simulink model "clusterDemo"  (Simulink 7.4)
settings: Solver=ode45  StartTime=0.0  StopTime=10.0  RelTol=1e-3
values from neighbouring files (symbols this model uses):
  A = 1    [clusterDemo.mat]
  B = [-1 -1 -1 -1 -1 -1 -1 -1 -1 -1 -1 -1 ... (21 elements, 1x21)]    [clusterDemo.mat]
  C = 1    [clusterDemo.mat]
  D = [0 0 0 0 0 0 0 0 0 0 0 0 ... (21 elements, 1x21)]    [clusterDemo.mat]
  N = 5    [clusterDemo.mat]    (also in firefliesDemo.mat = 10)
  var = 0    [clusterDemo.mat]    (also in firefliesDemo.mat = 3)
  x0 = 80    [clusterDemo.mat]
(part 2 of 4)

== system clusterDemo/Cluster/Cluster17 ==
  In1 : Inport  OutDataType=fixdt(1, 16)  OutScaling=2^0
  In2 : Inport  Port=2
  In3 : Inport  Port=3
  In4 : Inport  Port=4
  In5 : Inport  Port=5
  In6 : Inport  Port=6
  In7 : Inport  Port=7
  In8 : Inport  Port=8
  In9 : Inport  Port=9
  In10 : Inport  Port=10
  In11 : Inport  Port=11
  In12 : Inport  Port=12
  In13 : Inport  Port=13
  In14 : Inport  Port=14
  In15 : Inport  Port=15
  In16 : Inport  Port=16
  In17 : Inport  Port=17
  In18 : Inport  Port=18
  In19 : Inport  Port=19
  In20 : Inport  Port=20
  In21 : Inport  Port=21
  Mux : Mux  Inputs=21
  Scope1 : Scope
      settings: TimeRange=0.5847953216374258  YMin=-0.1657458563535892  YMax=1.21546961325967
  State-Space : StateSpace  A=A  B=B  C=C  D=D  X0=x0+var*rand(1)
  Out1 : Outport  OutDataType=fixdt(1, 16)  OutScaling=2^0
  wires:
  Mux/1 -> State-Space/1
  In1/1 -> Mux/1
  State-Space/1 -> Out1/1, Scope1/1
  In2/1 -> Mux/2
  In3/1 -> Mux/3
  In4/1 -> Mux/4
  In5/1 -> Mux/5
  In6/1 -> Mux/6
  In7/1 -> Mux/7
  In8/1 -> Mux/8
  In9/1 -> Mux/9
  In10/1 -> Mux/10
  In11/1 -> Mux/11
  In12/1 -> Mux/12
  In13/1 -> Mux/13
  In14/1 -> Mux/14
  In15/1 -> Mux/15
  In16/1 -> Mux/16
  In17/1 -> Mux/17
  In18/1 -> Mux/18
  In19/1 -> Mux/19
  In20/1 -> Mux/20
  In21/1 -> Mux/21

== system clusterDemo/Cluster/Cluster18 ==
  In1 : Inport  OutDataType=fixdt(1, 16)  OutScaling=2^0
  In2 : Inport  Port=2
  In3 : Inport  Port=3
  In4 : Inport  Port=4
  In5 : Inport  Port=5
  In6 : Inport  Port=6
  In7 : Inport  Port=7
  In8 : Inport  Port=8
  In9 : Inport  Port=9
  In10 : Inport  Port=10
  In11 : Inport  Port=11
  In12 : Inport  Port=12
  In13 : Inport  Port=13
  In14 : Inport  Port=14
  In15 : Inport  Port=15
  In16 : Inport  Port=16
  In17 : Inport  Port=17
  In18 : Inport  Port=18
  In19 : Inport  Port=19
  In20 : Inport  Port=20
  In21 : Inport  Port=21
  Mux : Mux  Inputs=21
  Scope1 : Scope
      settings: TimeRange=0.5847953216374258  YMin=-0.1657458563535892  YMax=1.21546961325967
  State-Space : StateSpace  A=A  B=B  C=C  D=D  X0=x0+var*rand(1)
  Out1 : Outport  OutDataType=fixdt(1, 16)  OutScaling=2^0
  wires:
  Mux/1 -> State-Space/1
  In1/1 -> Mux/1
  State-Space/1 -> Out1/1, Scope1/1
  In2/1 -> Mux/2
  In3/1 -> Mux/3
  In4/1 -> Mux/4
  In5/1 -> Mux/5
  In6/1 -> Mux/6
  In7/1 -> Mux/7
  In8/1 -> Mux/8
  In9/1 -> Mux/9
  In10/1 -> Mux/10
  In11/1 -> Mux/11
  In12/1 -> Mux/12
  In13/1 -> Mux/13
  In14/1 -> Mux/14
  In15/1 -> Mux/15
  In16/1 -> Mux/16
  In17/1 -> Mux/17
  In18/1 -> Mux/18
  In19/1 -> Mux/19
  In20/1 -> Mux/20
  In21/1 -> Mux/21

== system clusterDemo/Cluster/Cluster19 ==
  In1 : Inport  OutDataType=fixdt(1, 16)  OutScaling=2^0
  In2 : Inport  Port=2
  In3 : Inport  Port=3
  In4 : Inport  Port=4
  In5 : Inport  Port=5
  In6 : Inport  Port=6
  In7 : Inport  Port=7
  In8 : Inport  Port=8
  In9 : Inport  Port=9
  In10 : Inport  Port=10
  In11 : Inport  Port=11
  In12 : Inport  Port=12
  In13 : Inport  Port=13
  In14 : Inport  Port=14
  In15 : Inport  Port=15
  In16 : Inport  Port=16
  In17 : Inport  Port=17
  In18 : Inport  Port=18
  In19 : Inport  Port=19
  In20 : Inport  Port=20
  In21 : Inport  Port=21
  Mux : Mux  Inputs=21
  Scope1 : Scope
      settings: TimeRange=0.5847953216374258  YMin=-0.1657458563535892  YMax=1.21546961325967
  State-Space : StateSpace  A=A  B=B  C=C  D=D  X0=x0+var*rand(1)
  Out1 : Outport  OutDataType=fixdt(1, 16)  OutScaling=2^0
  wires:
  Mux/1 -> State-Space/1
  In1/1 -> Mux/1
  State-Space/1 -> Out1/1, Scope1/1
  In2/1 -> Mux/2
  In3/1 -> Mux/3
  In4/1 -> Mux/4
  In5/1 -> Mux/5
  In6/1 -> Mux/6
  In7/1 -> Mux/7
  In8/1 -> Mux/8
  In9/1 -> Mux/9
  In10/1 -> Mux/10
  In11/1 -> Mux/11
  In12/1 -> Mux/12
  In13/1 -> Mux/13
  In14/1 -> Mux/14
  In15/1 -> Mux/15
  In16/1 -> Mux/16
  In17/1 -> Mux/17
  In18/1 -> Mux/18
  In19/1 -> Mux/19
  In20/1 -> Mux/20
  In21/1 -> Mux/21

== system clusterDemo/Cluster/Cluster2 ==
  In1 : Inport  OutDataType=fixdt(1, 16)  OutScaling=2^0
  In2 : Inport  Port=2
  In3 : Inport  Port=3
  In4 : Inport  Port=4
  In5 : Inport  Port=5
  In6 : Inport  Port=6
  In7 : Inport  Port=7
  In8 : Inport  Port=8
  In9 : Inport  Port=9
  In10 : Inport  Port=10
  In11 : Inport  Port=11
  In12 : Inport  Port=12
  In13 : Inport  Port=13
  In14 : Inport  Port=14
  In15 : Inport  Port=15
  In16 : Inport  Port=16
  In17 : Inport  Port=17
  In18 : Inport  Port=18
  In19 : Inport  Port=19
  In20 : Inport  Port=20
  In21 : Inport  Port=21
  Mux : Mux  Inputs=21
  Scope1 : Scope
      settings: TimeRange=0.5847953216374258  YMin=-0.1657458563535892  YMax=1.21546961325967
  State-Space : StateSpace  A=A  B=B  C=C  D=D  X0=x0+var*rand(1)
  Out1 : Outport  OutDataType=fixdt(1, 16)  OutScaling=2^0
  wires:
  Mux/1 -> State-Space/1
  In1/1 -> Mux/1
  State-Space/1 -> Out1/1, Scope1/1
  In2/1 -> Mux/2
  In3/1 -> Mux/3
  In4/1 -> Mux/4
  In5/1 -> Mux/5
  In6/1 -> Mux/6
  In7/1 -> Mux/7
  In8/1 -> Mux/8
  In9/1 -> Mux/9
  In10/1 -> Mux/10
  In11/1 -> Mux/11
  In12/1 -> Mux/12
  In13/1 -> Mux/13
  In14/1 -> Mux/14
  In15/1 -> Mux/15
  In16/1 -> Mux/16
  In17/1 -> Mux/17
  In18/1 -> Mux/18
  In19/1 -> Mux/19
  In20/1 -> Mux/20
  In21/1 -> Mux/21

== system clusterDemo/Cluster/Cluster3 ==
  In1 : Inport  OutDataType=fixdt(1, 16)  OutScaling=2^0
  In2 : Inport  Port=2
  In3 : Inport  Port=3
  In4 : Inport  Port=4
  In5 : Inport  Port=5
  In6 : Inport  Port=6
  In7 : Inport  Port=7
  In8 : Inport  Port=8
  In9 : Inport  Port=9
  In10 : Inport  Port=10
  In11 : Inport  Port=11
  In12 : Inport  Port=12
  In13 : Inport  Port=13
  In14 : Inport  Port=14
  In15 : Inport  Port=15
  In16 : Inport  Port=16
  In17 : Inport  Port=17
  In18 : Inport  Port=18
  In19 : Inport  Port=19
  In20 : Inport  Port=20
  In21 : Inport  Port=21
  Mux : Mux  Inputs=21
  Scope1 : Scope
      settings: TimeRange=0.5847953216374258  YMin=-0.1657458563535892  YMax=1.21546961325967
  State-Space : StateSpace  A=A  B=B  C=C  D=D  X0=x0+var*rand(1)
  Out1 : Outport  OutDataType=fixdt(1, 16)  OutScaling=2^0
  wires:
  Mux/1 -> State-Space/1
  In1/1 -> Mux/1
  State-Space/1 -> Out1/1, Scope1/1
  In2/1 -> Mux/2
  In3/1 -> Mux/3
  In4/1 -> Mux/4
  In5/1 -> Mux/5
  In6/1 -> Mux/6
  In7/1 -> Mux/7
  In8/1 -> Mux/8
  In9/1 -> Mux/9
  In10/1 -> Mux/10
  In11/1 -> Mux/11
  In12/1 -> Mux/12
  In13/1 -> Mux/13
  In14/1 -> Mux/14
  In15/1 -> Mux/15
  In16/1 -> Mux/16
  In17/1 -> Mux/17
  In18/1 -> Mux/18
  In19/1 -> Mux/19
  In20/1 -> Mux/20
  In21/1 -> Mux/21

== system clusterDemo/Cluster/Cluster4 ==
  In1 : Inport  OutDataType=fixdt(1, 16)  OutScaling=2^0
  In2 : Inport  Port=2
  In3 : Inport  Port=3
  In4 : Inport  Port=4
  In5 : Inport  Port=5
  In6 : Inport  Port=6
  In7 : Inport  Port=7
  In8 : Inport  Port=8
  In9 : Inport  Port=9
  In10 : Inport  Port=10
  In11 : Inport  Port=11
  In12 : Inport  Port=12
  In13 : Inport  Port=13
  In14 : Inport  Port=14
  In15 : Inport  Port=15
  In16 : Inport  Port=16
  In17 : Inport  Port=17
  In18 : Inport  Port=18
  In19 : Inport  Port=19
  In20 : Inport  Port=20
  In21 : Inport  Port=21
  Mux : Mux  Inputs=21
  Scope1 : Scope
      settings: TimeRange=0.5847953216374258  YMin=-0.1657458563535892  YMax=1.21546961325967
  State-Space : StateSpace  A=A  B=B  C=C  D=D  X0=x0+var*rand(1)
  Out1 : Outport  OutDataType=fixdt(1, 16)  OutScaling=2^0
  wires:
  Mux/1 -> State-Space/1
  In1/1 -> Mux/1
  State-Space/1 -> Out1/1, Scope1/1
  In2/1 -> Mux/2
  In3/1 -> Mux/3
  In4/1 -> Mux/4
  In5/1 -> Mux/5
  In6/1 -> Mux/6
  In7/1 -> Mux/7
  In8/1 -> Mux/8
  In9/1 -> Mux/9
  In10/1 -> Mux/10
  In11/1 -> Mux/11
  In12/1 -> Mux/12
  In13/1 -> Mux/13
  In14/1 -> Mux/14
  In15/1 -> Mux/15
  In16/1 -> Mux/16
  In17/1 -> Mux/17
  In18/1 -> Mux/18
  In19/1 -> Mux/19
  In20/1 -> Mux/20
  In21/1 -> Mux/21

== system clusterDemo/Cluster/Cluster5 ==
  In1 : Inport  OutDataType=fixdt(1, 16)  OutScaling=2^0
  In2 : Inport  Port=2
  In3 : Inport  Port=3
  In4 : Inport  Port=4
  In5 : Inport  Port=5
  In6 : Inport  Port=6
  In7 : Inport  Port=7
  In8 : Inport  Port=8
  In9 : Inport  Port=9
  In10 : Inport  Port=10
  In11 : Inport  Port=11
  In12 : Inport  Port=12
  In13 : Inport  Port=13
  In14 : Inport  Port=14
  In15 : Inport  Port=15
  In16 : Inport  Port=16
  In17 : Inport  Port=17
  In18 : Inport  Port=18
  In19 : Inport  Port=19
  In20 : Inport  Port=20
  In21 : Inport  Port=21
  Mux : Mux  Inputs=21
  Scope1 : Scope
      settings: TimeRange=0.5847953216374258  YMin=-0.1657458563535892  YMax=1.21546961325967
  State-Space : StateSpace  A=A  B=B  C=C  D=D  X0=x0+var*rand(1)
  Out1 : Outport  OutDataType=fixdt(1, 16)  OutScaling=2^0
  wires:
  Mux/1 -> State-Space/1
  In1/1 -> Mux/1
  State-Space/1 -> Out1/1, Scope1/1
  In2/1 -> Mux/2
  In3/1 -> Mux/3
  In4/1 -> Mux/4
  In5/1 -> Mux/5
  In6/1 -> Mux/6
  In7/1 -> Mux/7
  In8/1 -> Mux/8
  In9/1 -> Mux/9
  In10/1 -> Mux/10
  In11/1 -> Mux/11
  In12/1 -> Mux/12
  In13/1 -> Mux/13
  In14/1 -> Mux/14
  In15/1 -> Mux/15
  In16/1 -> Mux/16
  In17/1 -> Mux/17
  In18/1 -> Mux/18
  In19/1 -> Mux/19
  In20/1 -> Mux/20
  In21/1 -> Mux/21

== system clusterDemo/Cluster/Cluster6 ==
  In1 : Inport  OutDataType=fixdt(1, 16)  OutScaling=2^0
  In2 : Inport  Port=2
  In3 : Inport  Port=3
  In4 : Inport  Port=4
  In5 : Inport  Port=5
  In6 : Inport  Port=6
  In7 : Inport  Port=7
  In8 : Inport  Port=8
  In9 : Inport  Port=9
  In10 : Inport  Port=10
  In11 : Inport  Port=11
  In12 : Inport  Port=12
  In13 : Inport  Port=13
  In14 : Inport  Port=14
  In15 : Inport  Port=15
  In16 : Inport  Port=16
  In17 : Inport  Port=17
  In18 : Inport  Port=18
  In19 : Inport  Port=19
  In20 : Inport  Port=20
  In21 : Inport  Port=21
  Mux : Mux  Inputs=21
  Scope1 : Scope
      settings: TimeRange=0.5847953216374258  YMin=-0.1657458563535892  YMax=1.21546961325967
  State-Space : StateSpace  A=A  B=B  C=C  D=D  X0=x0+var*rand(1)
  Out1 : Outport  OutDataType=fixdt(1, 16)  OutScaling=2^0
  wires:
  Mux/1 -> State-Space/1
  In1/1 -> Mux/1
  State-Space/1 -> Out1/1, Scope1/1
  In2/1 -> Mux/2
  In3/1 -> Mux/3
  In4/1 -> Mux/4
  In5/1 -> Mux/5
  In6/1 -> Mux/6
  In7/1 -> Mux/7
  In8/1 -> Mux/8
  In9/1 -> Mux/9
  In10/1 -> Mux/10
  In11/1 -> Mux/11
  In12/1 -> Mux/12
  In13/1 -> Mux/13
  In14/1 -> Mux/14
  In15/1 -> Mux/15
  In16/1 -> Mux/16
  In17/1 -> Mux/17
  In18/1 -> Mux/18
  In19/1 -> Mux/19
  In20/1 -> Mux/20
  In21/1 -> Mux/21

== system clusterDemo/Cluster/Cluster7 ==
  In1 : Inport  OutDataType=fixdt(1, 16)  OutScaling=2^0
  In2 : Inport  Port=2
  In3 : Inport  Port=3
  In4 : Inport  Port=4
  In5 : Inport  Port=5
  In6 : Inport  Port=6
  In7 : Inport  Port=7
  In8 : Inport  Port=8
  In9 : Inport  Port=9
  In10 : Inport  Port=10
  In11 : Inport  Port=11
  In12 : Inport  Port=12
  In13 : Inport  Port=13
  In14 : Inport  Port=14
  In15 : Inport  Port=15
  In16 : Inport  Port=16
  In17 : Inport  Port=17
  In18 : Inport  Port=18
  In19 : Inport  Port=19
  In20 : Inport  Port=20
  In21 : Inport  Port=21
  Mux : Mux  Inputs=21
  Scope1 : Scope
      settings: TimeRange=0.5847953216374258  YMin=-0.1657458563535892  YMax=1.21546961325967
  State-Space : StateSpace  A=A  B=B  C=C  D=D  X0=x0+var*rand(1)
  Out1 : Outport  OutDataType=fixdt(1, 16)  OutScaling=2^0
  wires:
  Mux/1 -> State-Space/1
  In1/1 -> Mux/1
  State-Space/1 -> Out1/1, Scope1/1
  In2/1 -> Mux/2
  In3/1 -> Mux/3
  In4/1 -> Mux/4
  In5/1 -> Mux/5
  In6/1 -> Mux/6
  In7/1 -> Mux/7
  In8/1 -> Mux/8
  In9/1 -> Mux/9
  In10/1 -> Mux/10
  In11/1 -> Mux/11
  In12/1 -> Mux/12
  In13/1 -> Mux/13
  In14/1 -> Mux/14
  In15/1 -> Mux/15
  In16/1 -> Mux/16
  In17/1 -> Mux/17
  In18/1 -> Mux/18
  In19/1 -> Mux/19
  In20/1 -> Mux/20
  In21/1 -> Mux/21

== system clusterDemo/Cluster/Cluster8 ==
  In1 : Inport  OutDataType=fixdt(1, 16)  OutScaling=2^0
  In2 : Inport  Port=2
  In3 : Inport  Port=3
  In4 : Inport  Port=4
  In5 : Inport  Port=5
  In6 : Inport  Port=6
  In7 : Inport  Port=7
  In8 : Inport  Port=8
  In9 : Inport  Port=9
  In10 : Inport  Port=10
  In11 : Inport  Port=11
  In12 : Inport  Port=12
  In13 : Inport  Port=13
  In14 : Inport  Port=14
  In15 : Inport  Port=15
  In16 : Inport  Port=16
  In17 : Inport  Port=17
  In18 : Inport  Port=18
  In19 : Inport  Port=19
  In20 : Inport  Port=20
  In21 : Inport  Port=21
  Mux : Mux  Inputs=21
  Scope1 : Scope
      settings: TimeRange=0.5847953216374258  YMin=-0.1657458563535892  YMax=1.21546961325967
  State-Space : StateSpace  A=A  B=B  C=C  D=D  X0=x0+var*rand(1)
  Out1 : Outport  OutDataType=fixdt(1, 16)  OutScaling=2^0
  wires:
  Mux/1 -> State-Space/1
  In1/1 -> Mux/1
  State-Space/1 -> Out1/1, Scope1/1
  In2/1 -> Mux/2
  In3/1 -> Mux/3
  In4/1 -> Mux/4
  In5/1 -> Mux/5
  In6/1 -> Mux/6
  In7/1 -> Mux/7
  In8/1 -> Mux/8
  In9/1 -> Mux/9
  In10/1 -> Mux/10
  In11/1 -> Mux/11
  In12/1 -> Mux/12
  In13/1 -> Mux/13
  In14/1 -> Mux/14
  In15/1 -> Mux/15
  In16/1 -> Mux/16
  In17/1 -> Mux/17
  In18/1 -> Mux/18
  In19/1 -> Mux/19
  In20/1 -> Mux/20
  In21/1 -> Mux/21

== system clusterDemo/Cluster/Cluster9 ==
  In1 : Inport  OutDataType=fixdt(1, 16)  OutScaling=2^0
  In2 : Inport  Port=2
  In3 : Inport  Port=3
  In4 : Inport  Port=4
  In5 : Inport  Port=5
  In6 : Inport  Port=6
  In7 : Inport  Port=7
  In8 : Inport  Port=8
  In9 : Inport  Port=9
  In10 : Inport  Port=10
  In11 : Inport  Port=11
  In12 : Inport  Port=12
  In13 : Inport  Port=13
  In14 : Inport  Port=14
  In15 : Inport  Port=15
  In16 : Inport  Port=16
  In17 : Inport  Port=17
  In18 : Inport  Port=18
  In19 : Inport  Port=19
  In20 : Inport  Port=20
  In21 : Inport  Port=21
  Mux : Mux  Inputs=21
  Scope1 : Scope
      settings: TimeRange=0.5847953216374258  YMin=-0.1657458563535892  YMax=1.21546961325967
  State-Space : StateSpace  A=A  B=B  C=C  D=D  X0=x0+var*rand(1)
  Out1 : Outport  OutDataType=fixdt(1, 16)  OutScaling=2^0
  wires:
  Mux/1 -> State-Space/1
  In1/1 -> Mux/1
  State-Space/1 -> Out1/1, Scope1/1
  In2/1 -> Mux/2
  In3/1 -> Mux/3
  In4/1 -> Mux/4
  In5/1 -> Mux/5
  In6/1 -> Mux/6
  In7/1 -> Mux/7
  In8/1 -> Mux/8
  In9/1 -> Mux/9
  In10/1 -> Mux/10
  In11/1 -> Mux/11
  In12/1 -> Mux/12
  In13/1 -> Mux/13
  In14/1 -> Mux/14
  In15/1 -> Mux/15
  In16/1 -> Mux/16
  In17/1 -> Mux/17
  In18/1 -> Mux/18
  In19/1 -> Mux/19
  In20/1 -> Mux/20
  In21/1 -> Mux/21

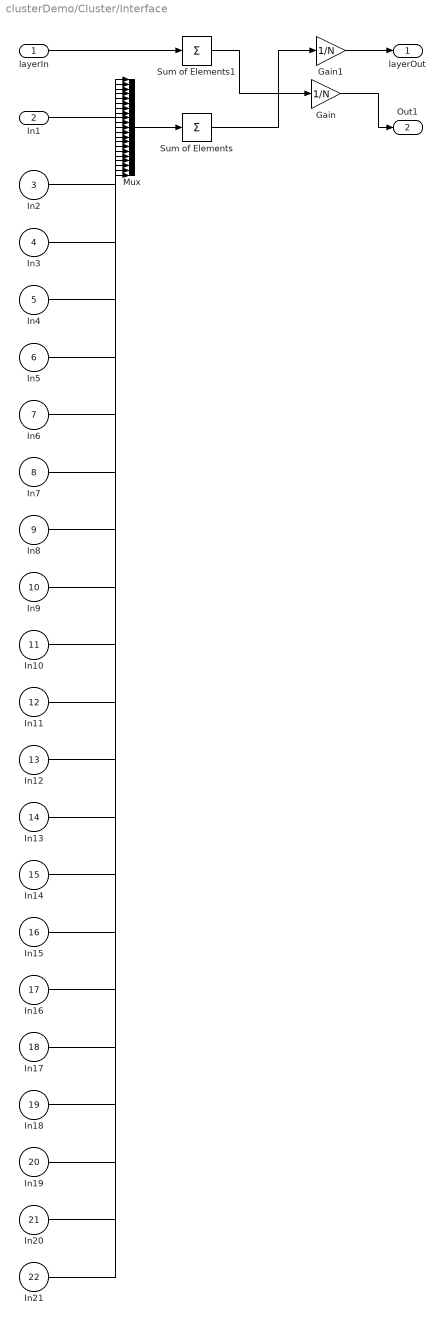
== system clusterDemo/Cluster/Interface ==
  layerIn : Inport  OutDataType=fixdt(1, 16)  OutScaling=2^0
  In1 : Inport  Port=2  OutDataType=fixdt(1, 16)  OutScaling=2^0
  In2 : Inport  Port=3
  In3 : Inport  Port=4
  In4 : Inport  Port=5
  In5 : Inport  Port=6
  In6 : Inport  Port=7
  In7 : Inport  Port=8
  In8 : Inport  Port=9
  In9 : Inport  Port=10
  In10 : Inport  Port=11
  In11 : Inport  Port=12
  In12 : Inport  Port=13
  In13 : Inport  Port=14
  In14 : Inport  Port=15
  In15 : Inport  Port=16
  In16 : Inport  Port=17
  In17 : Inport  Port=18
  In18 : Inport  Port=19
  In19 : Inport  Port=20
  In20 : Inport  Port=21
  In21 : Inport  Port=22
  Gain : Gain  Gain=1/N  ParameterDataType=fixdt(1, 16)  ParameterScaling=2^0  OutDataType=fixdt(1, 16)  OutScaling=2^0
  Gain1 : Gain  Gain=1/N  ParameterDataType=fixdt(1, 16)  ParameterScaling=2^0  OutDataType=fixdt(1, 16)  OutScaling=2^0
  Mux : Mux  Inputs=21
  Sum of Elements : Sum  Inputs=+  OutDataType=fixdt(1, 16)  OutScaling=2^-10
  Sum of Elements1 : Sum  Inputs=+  OutDataType=fixdt(1, 16)  OutScaling=2^-10
  layerOut : Outport  OutDataType=fixdt(1, 16)  OutScaling=2^0
  Out1 : Outport  Port=2  OutDataType=fixdt(1, 16)  OutScaling=2^0
  wires:
  Mux/1 -> Sum of Elements/1
  In1/1 -> Mux/1
  Sum of Elements/1 -> Gain1/1
  layerIn/1 -> Sum of Elements1/1
  Sum of Elements1/1 -> Gain/1
  Gain/1 -> Out1/1
  Gain1/1 -> layerOut/1
  In2/1 -> Mux/2
  In3/1 -> Mux/3
  In4/1 -> Mux/4
  In5/1 -> Mux/5
  In6/1 -> Mux/6
  In7/1 -> Mux/7
  In8/1 -> Mux/8
  In9/1 -> Mux/9
  In10/1 -> Mux/10
  In11/1 -> Mux/11
  In12/1 -> Mux/12
  In13/1 -> Mux/13
  In14/1 -> Mux/14
  In15/1 -> Mux/15
  In16/1 -> Mux/16
  In17/1 -> Mux/17
  In18/1 -> Mux/18
  In19/1 -> Mux/19
  In20/1 -> Mux/20
  In21/1 -> Mux/21

== system clusterDemo/Cluster1/Cluster ==
  In1 : Inport  OutDataType=fixdt(1, 16)  OutScaling=2^0
  In2 : Inport  Port=2
  In3 : Inport  Port=3
  In4 : Inport  Port=4
  In5 : Inport  Port=5
  In6 : Inport  Port=6
  In7 : Inport  Port=7
  In8 : Inport  Port=8
  In9 : Inport  Port=9
  In10 : Inport  Port=10
  In11 : Inport  Port=11
  In12 : Inport  Port=12
  In13 : Inport  Port=13
  In14 : Inport  Port=14
  In15 : Inport  Port=15
  In16 : Inport  Port=16
  In17 : Inport  Port=17
  In18 : Inport  Port=18
  In19 : Inport  Port=19
  In20 : Inport  Port=20
  In21 : Inport  Port=21
  Mux : Mux  Inputs=21
  Scope1 : Scope
      settings: TimeRange=0.5847953216374258  YMin=-0.1657458563535892  YMax=1.21546961325967
  State-Space : StateSpace  A=A  B=B  C=C  D=D  X0=x0+var*rand(1)
  Out1 : Outport  OutDataType=fixdt(1, 16)  OutScaling=2^0
  wires:
  Mux/1 -> State-Space/1
  In1/1 -> Mux/1
  State-Space/1 -> Out1/1, Scope1/1
  In2/1 -> Mux/2
  In3/1 -> Mux/3
  In4/1 -> Mux/4
  In5/1 -> Mux/5
  In6/1 -> Mux/6
  In7/1 -> Mux/7
  In8/1 -> Mux/8
  In9/1 -> Mux/9
  In10/1 -> Mux/10
  In11/1 -> Mux/11
  In12/1 -> Mux/12
  In13/1 -> Mux/13
  In14/1 -> Mux/14
  In15/1 -> Mux/15
  In16/1 -> Mux/16
  In17/1 -> Mux/17
  In18/1 -> Mux/18
  In19/1 -> Mux/19
  In20/1 -> Mux/20
  In21/1 -> Mux/21

== system clusterDemo/Cluster1/Cluster1 ==
  In1 : Inport  OutDataType=fixdt(1, 16)  OutScaling=2^0
  In2 : Inport  Port=2
  In3 : Inport  Port=3
  In4 : Inport  Port=4
  In5 : Inport  Port=5
  In6 : Inport  Port=6
  In7 : Inport  Port=7
  In8 : Inport  Port=8
  In9 : Inport  Port=9
  In10 : Inport  Port=10
  In11 : Inport  Port=11
  In12 : Inport  Port=12
  In13 : Inport  Port=13
  In14 : Inport  Port=14
  In15 : Inport  Port=15
  In16 : Inport  Port=16
  In17 : Inport  Port=17
  In18 : Inport  Port=18
  In19 : Inport  Port=19
  In20 : Inport  Port=20
  In21 : Inport  Port=21
  Mux : Mux  Inputs=21
  Scope1 : Scope
      settings: TimeRange=0.5847953216374258  YMin=-0.1657458563535892  YMax=1.21546961325967
  State-Space : StateSpace  A=A  B=B  C=C  D=D  X0=x0+var*rand(1)
  Out1 : Outport  OutDataType=fixdt(1, 16)  OutScaling=2^0
  wires:
  Mux/1 -> State-Space/1
  In1/1 -> Mux/1
  State-Space/1 -> Out1/1, Scope1/1
  In2/1 -> Mux/2
  In3/1 -> Mux/3
  In4/1 -> Mux/4
  In5/1 -> Mux/5
  In6/1 -> Mux/6
  In7/1 -> Mux/7
  In8/1 -> Mux/8
  In9/1 -> Mux/9
  In10/1 -> Mux/10
  In11/1 -> Mux/11
  In12/1 -> Mux/12
  In13/1 -> Mux/13
  In14/1 -> Mux/14
  In15/1 -> Mux/15
  In16/1 -> Mux/16
  In17/1 -> Mux/17
  In18/1 -> Mux/18
  In19/1 -> Mux/19
  In20/1 -> Mux/20
  In21/1 -> Mux/21

== system clusterDemo/Cluster1/Cluster10 ==
  In1 : Inport  OutDataType=fixdt(1, 16)  OutScaling=2^0
  In2 : Inport  Port=2
  In3 : Inport  Port=3
  In4 : Inport  Port=4
  In5 : Inport  Port=5
  In6 : Inport  Port=6
  In7 : Inport  Port=7
  In8 : Inport  Port=8
  In9 : Inport  Port=9
  In10 : Inport  Port=10
  In11 : Inport  Port=11
  In12 : Inport  Port=12
  In13 : Inport  Port=13
  In14 : Inport  Port=14
  In15 : Inport  Port=15
  In16 : Inport  Port=16
  In17 : Inport  Port=17
  In18 : Inport  Port=18
  In19 : Inport  Port=19
  In20 : Inport  Port=20
  In21 : Inport  Port=21
  Mux : Mux  Inputs=21
  Scope1 : Scope
      settings: TimeRange=0.5847953216374258  YMin=-0.1657458563535892  YMax=1.21546961325967
  State-Space : StateSpace  A=A  B=B  C=C  D=D  X0=x0+var*rand(1)
  Out1 : Outport  OutDataType=fixdt(1, 16)  OutScaling=2^0
  wires:
  Mux/1 -> State-Space/1
  In1/1 -> Mux/1
  State-Space/1 -> Out1/1, Scope1/1
  In2/1 -> Mux/2
  In3/1 -> Mux/3
  In4/1 -> Mux/4
  In5/1 -> Mux/5
  In6/1 -> Mux/6
  In7/1 -> Mux/7
  In8/1 -> Mux/8
  In9/1 -> Mux/9
  In10/1 -> Mux/10
  In11/1 -> Mux/11
  In12/1 -> Mux/12
  In13/1 -> Mux/13
  In14/1 -> Mux/14
  In15/1 -> Mux/15
  In16/1 -> Mux/16
  In17/1 -> Mux/17
  In18/1 -> Mux/18
  In19/1 -> Mux/19
  In20/1 -> Mux/20
  In21/1 -> Mux/21

== system clusterDemo/Cluster1/Cluster11 ==
  In1 : Inport  OutDataType=fixdt(1, 16)  OutScaling=2^0
  In2 : Inport  Port=2
  In3 : Inport  Port=3
  In4 : Inport  Port=4
  In5 : Inport  Port=5
  In6 : Inport  Port=6
  In7 : Inport  Port=7
  In8 : Inport  Port=8
  In9 : Inport  Port=9
  In10 : Inport  Port=10
  In11 : Inport  Port=11
  In12 : Inport  Port=12
  In13 : Inport  Port=13
  In14 : Inport  Port=14
  In15 : Inport  Port=15
  In16 : Inport  Port=16
  In17 : Inport  Port=17
  In18 : Inport  Port=18
  In19 : Inport  Port=19
  In20 : Inport  Port=20
  In21 : Inport  Port=21
  Mux : Mux  Inputs=21
  Scope1 : Scope
      settings: TimeRange=0.5847953216374258  YMin=-0.1657458563535892  YMax=1.21546961325967
  State-Space : StateSpace  A=A  B=B  C=C  D=D  X0=x0+var*rand(1)
  Out1 : Outport  OutDataType=fixdt(1, 16)  OutScaling=2^0
  wires:
  Mux/1 -> State-Space/1
  In1/1 -> Mux/1
  State-Space/1 -> Out1/1, Scope1/1
  In2/1 -> Mux/2
  In3/1 -> Mux/3
  In4/1 -> Mux/4
  In5/1 -> Mux/5
  In6/1 -> Mux/6
  In7/1 -> Mux/7
  In8/1 -> Mux/8
  In9/1 -> Mux/9
  In10/1 -> Mux/10
  In11/1 -> Mux/11
  In12/1 -> Mux/12
  In13/1 -> Mux/13
  In14/1 -> Mux/14
  In15/1 -> Mux/15
  In16/1 -> Mux/16
  In17/1 -> Mux/17
  In18/1 -> Mux/18
  In19/1 -> Mux/19
  In20/1 -> Mux/20
  In21/1 -> Mux/21

== system clusterDemo/Cluster1/Cluster12 ==
  In1 : Inport  OutDataType=fixdt(1, 16)  OutScaling=2^0
  In2 : Inport  Port=2
  In3 : Inport  Port=3
  In4 : Inport  Port=4
  In5 : Inport  Port=5
  In6 : Inport  Port=6
  In7 : Inport  Port=7
  In8 : Inport  Port=8
  In9 : Inport  Port=9
  In10 : Inport  Port=10
  In11 : Inport  Port=11
  In12 : Inport  Port=12
  In13 : Inport  Port=13
  In14 : Inport  Port=14
  In15 : Inport  Port=15
  In16 : Inport  Port=16
  In17 : Inport  Port=17
  In18 : Inport  Port=18
  In19 : Inport  Port=19
  In20 : Inport  Port=20
  In21 : Inport  Port=21
  Mux : Mux  Inputs=21
  Scope1 : Scope
      settings: TimeRange=0.5847953216374258  YMin=-0.1657458563535892  YMax=1.21546961325967
  State-Space : StateSpace  A=A  B=B  C=C  D=D  X0=x0+var*rand(1)
  Out1 : Outport  OutDataType=fixdt(1, 16)  OutScaling=2^0
  wires:
  Mux/1 -> State-Space/1
  In1/1 -> Mux/1
  State-Space/1 -> Out1/1, Scope1/1
  In2/1 -> Mux/2
  In3/1 -> Mux/3
  In4/1 -> Mux/4
  In5/1 -> Mux/5
  In6/1 -> Mux/6
  In7/1 -> Mux/7
  In8/1 -> Mux/8
  In9/1 -> Mux/9
  In10/1 -> Mux/10
  In11/1 -> Mux/11
  In12/1 -> Mux/12
  In13/1 -> Mux/13
  In14/1 -> Mux/14
  In15/1 -> Mux/15
  In16/1 -> Mux/16
  In17/1 -> Mux/17
  In18/1 -> Mux/18
  In19/1 -> Mux/19
  In20/1 -> Mux/20
  In21/1 -> Mux/21

== system clusterDemo/Cluster1/Cluster13 ==
  In1 : Inport  OutDataType=fixdt(1, 16)  OutScaling=2^0
  In2 : Inport  Port=2
  In3 : Inport  Port=3
  In4 : Inport  Port=4
  In5 : Inport  Port=5
  In6 : Inport  Port=6
  In7 : Inport  Port=7
  In8 : Inport  Port=8
  In9 : Inport  Port=9
  In10 : Inport  Port=10
  In11 : Inport  Port=11
  In12 : Inport  Port=12
  In13 : Inport  Port=13
  In14 : Inport  Port=14
  In15 : Inport  Port=15
  In16 : Inport  Port=16
  In17 : Inport  Port=17
  In18 : Inport  Port=18
  In19 : Inport  Port=19
  In20 : Inport  Port=20
  In21 : Inport  Port=21
  Mux : Mux  Inputs=21
  Scope1 : Scope
      settings: TimeRange=0.5847953216374258  YMin=-0.1657458563535892  YMax=1.21546961325967
  State-Space : StateSpace  A=A  B=B  C=C  D=D  X0=x0+var*rand(1)
  Out1 : Outport  OutDataType=fixdt(1, 16)  OutScaling=2^0
  wires:
  Mux/1 -> State-Space/1
  In1/1 -> Mux/1
  State-Space/1 -> Out1/1, Scope1/1
  In2/1 -> Mux/2
  In3/1 -> Mux/3
  In4/1 -> Mux/4
  In5/1 -> Mux/5
  In6/1 -> Mux/6
  In7/1 -> Mux/7
  In8/1 -> Mux/8
  In9/1 -> Mux/9
  In10/1 -> Mux/10
  In11/1 -> Mux/11
  In12/1 -> Mux/12
  In13/1 -> Mux/13
  In14/1 -> Mux/14
  In15/1 -> Mux/15
  In16/1 -> Mux/16
  In17/1 -> Mux/17
  In18/1 -> Mux/18
  In19/1 -> Mux/19
  In20/1 -> Mux/20
  In21/1 -> Mux/21

== system clusterDemo/Cluster1/Cluster14 ==
  In1 : Inport  OutDataType=fixdt(1, 16)  OutScaling=2^0
  In2 : Inport  Port=2
  In3 : Inport  Port=3
  In4 : Inport  Port=4
  In5 : Inport  Port=5
  In6 : Inport  Port=6
  In7 : Inport  Port=7
  In8 : Inport  Port=8
  In9 : Inport  Port=9
  In10 : Inport  Port=10
  In11 : Inport  Port=11
  In12 : Inport  Port=12
  In13 : Inport  Port=13
  In14 : Inport  Port=14
  In15 : Inport  Port=15
  In16 : Inport  Port=16
  In17 : Inport  Port=17
  In18 : Inport  Port=18
  In19 : Inport  Port=19
  In20 : Inport  Port=20
  In21 : Inport  Port=21
  Mux : Mux  Inputs=21
  Scope1 : Scope
      settings: TimeRange=0.5847953216374258  YMin=-0.1657458563535892  YMax=1.21546961325967
  State-Space : StateSpace  A=A  B=B  C=C  D=D  X0=x0+var*rand(1)
  Out1 : Outport  OutDataType=fixdt(1, 16)  OutScaling=2^0
  wires:
  Mux/1 -> State-Space/1
  In1/1 -> Mux/1
  State-Space/1 -> Out1/1, Scope1/1
  In2/1 -> Mux/2
  In3/1 -> Mux/3
  In4/1 -> Mux/4
  In5/1 -> Mux/5
  In6/1 -> Mux/6
  In7/1 -> Mux/7
  In8/1 -> Mux/8
  In9/1 -> Mux/9
  In10/1 -> Mux/10
  In11/1 -> Mux/11
  In12/1 -> Mux/12
  In13/1 -> Mux/13
  In14/1 -> Mux/14
  In15/1 -> Mux/15
  In16/1 -> Mux/16
  In17/1 -> Mux/17
  In18/1 -> Mux/18
  In19/1 -> Mux/19
  In20/1 -> Mux/20
  In21/1 -> Mux/21

== system clusterDemo/Cluster1/Cluster15 ==
  In1 : Inport  OutDataType=fixdt(1, 16)  OutScaling=2^0
  In2 : Inport  Port=2
  In3 : Inport  Port=3
  In4 : Inport  Port=4
  In5 : Inport  Port=5
  In6 : Inport  Port=6
  In7 : Inport  Port=7
  In8 : Inport  Port=8
  In9 : Inport  Port=9
  In10 : Inport  Port=10
  In11 : Inport  Port=11
  In12 : Inport  Port=12
  In13 : Inport  Port=13
  In14 : Inport  Port=14
  In15 : Inport  Port=15
  In16 : Inport  Port=16
  In17 : Inport  Port=17
  In18 : Inport  Port=18
  In19 : Inport  Port=19
  In20 : Inport  Port=20
  In21 : Inport  Port=21
  Mux : Mux  Inputs=21
  Scope1 : Scope
      settings: TimeRange=0.5847953216374258  YMin=-0.1657458563535892  YMax=1.21546961325967
  State-Space : StateSpace  A=A  B=B  C=C  D=D  X0=x0+var*rand(1)
  Out1 : Outport  OutDataType=fixdt(1, 16)  OutScaling=2^0
  wires:
  Mux/1 -> State-Space/1
  In1/1 -> Mux/1
  State-Space/1 -> Out1/1, Scope1/1
  In2/1 -> Mux/2
  In3/1 -> Mux/3
  In4/1 -> Mux/4
  In5/1 -> Mux/5
  In6/1 -> Mux/6
  In7/1 -> Mux/7
  In8/1 -> Mux/8
  In9/1 -> Mux/9
  In10/1 -> Mux/10
  In11/1 -> Mux/11
  In12/1 -> Mux/12
  In13/1 -> Mux/13
  In14/1 -> Mux/14
  In15/1 -> Mux/15
  In16/1 -> Mux/16
  In17/1 -> Mux/17
  In18/1 -> Mux/18
  In19/1 -> Mux/19
  In20/1 -> Mux/20
  In21/1 -> Mux/21

== system clusterDemo/Cluster1/Cluster16 ==
  In1 : Inport  OutDataType=fixdt(1, 16)  OutScaling=2^0
  In2 : Inport  Port=2
  In3 : Inport  Port=3
  In4 : Inport  Port=4
  In5 : Inport  Port=5
  In6 : Inport  Port=6
  In7 : Inport  Port=7
  In8 : Inport  Port=8
  In9 : Inport  Port=9
  In10 : Inport  Port=10
  In11 : Inport  Port=11
  In12 : Inport  Port=12
  In13 : Inport  Port=13
  In14 : Inport  Port=14
  In15 : Inport  Port=15
  In16 : Inport  Port=16
  In17 : Inport  Port=17
  In18 : Inport  Port=18
  In19 : Inport  Port=19
  In20 : Inport  Port=20
  In21 : Inport  Port=21
  Mux : Mux  Inputs=21
  Scope1 : Scope
      settings: TimeRange=0.5847953216374258  YMin=-0.1657458563535892  YMax=1.21546961325967
  State-Space : StateSpace  A=A  B=B  C=C  D=D  X0=x0+var*rand(1)
  Out1 : Outport  OutDataType=fixdt(1, 16)  OutScaling=2^0
  wires:
  Mux/1 -> State-Space/1
  In1/1 -> Mux/1
  State-Space/1 -> Out1/1, Scope1/1
  In2/1 -> Mux/2
  In3/1 -> Mux/3
  In4/1 -> Mux/4
  In5/1 -> Mux/5
  In6/1 -> Mux/6
  In7/1 -> Mux/7
  In8/1 -> Mux/8
  In9/1 -> Mux/9
  In10/1 -> Mux/10
  In11/1 -> Mux/11
  In12/1 -> Mux/12
  In13/1 -> Mux/13
  In14/1 -> Mux/14
  In15/1 -> Mux/15
  In16/1 -> Mux/16
  In17/1 -> Mux/17
  In18/1 -> Mux/18
  In19/1 -> Mux/19
  In20/1 -> Mux/20
  In21/1 -> Mux/21

== system clusterDemo/Cluster1/Cluster17 ==
  In1 : Inport  OutDataType=fixdt(1, 16)  OutScaling=2^0
  In2 : Inport  Port=2
  In3 : Inport  Port=3
  In4 : Inport  Port=4
  In5 : Inport  Port=5
  In6 : Inport  Port=6
  In7 : Inport  Port=7
  In8 : Inport  Port=8
  In9 : Inport  Port=9
  In10 : Inport  Port=10
  In11 : Inport  Port=11
  In12 : Inport  Port=12
  In13 : Inport  Port=13
  In14 : Inport  Port=14
  In15 : Inport  Port=15
  In16 : Inport  Port=16
  In17 : Inport  Port=17
  In18 : Inport  Port=18
  In19 : Inport  Port=19
  In20 : Inport  Port=20
  In21 : Inport  Port=21
  Mux : Mux  Inputs=21
  Scope1 : Scope
      settings: TimeRange=0.5847953216374258  YMin=-0.1657458563535892  YMax=1.21546961325967
  State-Space : StateSpace  A=A  B=B  C=C  D=D  X0=x0+var*rand(1)
  Out1 : Outport  OutDataType=fixdt(1, 16)  OutScaling=2^0
  wires:
  Mux/1 -> State-Space/1
  In1/1 -> Mux/1
  State-Space/1 -> Out1/1, Scope1/1
  In2/1 -> Mux/2
  In3/1 -> Mux/3
  In4/1 -> Mux/4
  In5/1 -> Mux/5
  In6/1 -> Mux/6
  In7/1 -> Mux/7
  In8/1 -> Mux/8
  In9/1 -> Mux/9
  In10/1 -> Mux/10
  In11/1 -> Mux/11
  In12/1 -> Mux/12
  In13/1 -> Mux/13
  In14/1 -> Mux/14
  In15/1 -> Mux/15
  In16/1 -> Mux/16
  In17/1 -> Mux/17
  In18/1 -> Mux/18
  In19/1 -> Mux/19
  In20/1 -> Mux/20
  In21/1 -> Mux/21

== system clusterDemo/Cluster1/Cluster18 ==
  In1 : Inport  OutDataType=fixdt(1, 16)  OutScaling=2^0
  In2 : Inport  Port=2
  In3 : Inport  Port=3
  In4 : Inport  Port=4
  In5 : Inport  Port=5
  In6 : Inport  Port=6
  In7 : Inport  Port=7
  In8 : Inport  Port=8
  In9 : Inport  Port=9
  In10 : Inport  Port=10
  In11 : Inport  Port=11
  In12 : Inport  Port=12
  In13 : Inport  Port=13
  In14 : Inport  Port=14
  In15 : Inport  Port=15
  In16 : Inport  Port=16
  In17 : Inport  Port=17
  In18 : Inport  Port=18
  In19 : Inport  Port=19
  In20 : Inport  Port=20
  In21 : Inport  Port=21
  Mux : Mux  Inputs=21
  Scope1 : Scope
      settings: TimeRange=0.5847953216374258  YMin=-0.1657458563535892  YMax=1.21546961325967
  State-Space : StateSpace  A=A  B=B  C=C  D=D  X0=x0+var*rand(1)
  Out1 : Outport  OutDataType=fixdt(1, 16)  OutScaling=2^0
  wires:
  Mux/1 -> State-Space/1
  In1/1 -> Mux/1
  State-Space/1 -> Out1/1, Scope1/1
  In2/1 -> Mux/2
  In3/1 -> Mux/3
  In4/1 -> Mux/4
  In5/1 -> Mux/5
  In6/1 -> Mux/6
  In7/1 -> Mux/7
  In8/1 -> Mux/8
  In9/1 -> Mux/9
  In10/1 -> Mux/10
  In11/1 -> Mux/11
  In12/1 -> Mux/12
  In13/1 -> Mux/13
  In14/1 -> Mux/14
  In15/1 -> Mux/15
  In16/1 -> Mux/16
  In17/1 -> Mux/17
  In18/1 -> Mux/18
  In19/1 -> Mux/19
  In20/1 -> Mux/20
  In21/1 -> Mux/21

== system clusterDemo/Cluster1/Cluster19 ==
  In1 : Inport  OutDataType=fixdt(1, 16)  OutScaling=2^0
  In2 : Inport  Port=2
  In3 : Inport  Port=3
  In4 : Inport  Port=4
  In5 : Inport  Port=5
  In6 : Inport  Port=6
  In7 : Inport  Port=7
  In8 : Inport  Port=8
  In9 : Inport  Port=9
  In10 : Inport  Port=10
  In11 : Inport  Port=11
  In12 : Inport  Port=12
  In13 : Inport  Port=13
  In14 : Inport  Port=14
  In15 : Inport  Port=15
  In16 : Inport  Port=16
  In17 : Inport  Port=17
  In18 : Inport  Port=18
  In19 : Inport  Port=19
  In20 : Inport  Port=20
  In21 : Inport  Port=21
  Mux : Mux  Inputs=21
  Scope1 : Scope
      settings: TimeRange=0.5847953216374258  YMin=-0.1657458563535892  YMax=1.21546961325967
  State-Space : StateSpace  A=A  B=B  C=C  D=D  X0=x0+var*rand(1)
  Out1 : Outport  OutDataType=fixdt(1, 16)  OutScaling=2^0
  wires:
  Mux/1 -> State-Space/1
  In1/1 -> Mux/1
  State-Space/1 -> Out1/1, Scope1/1
  In2/1 -> Mux/2
  In3/1 -> Mux/3
  In4/1 -> Mux/4
  In5/1 -> Mux/5
  In6/1 -> Mux/6
  In7/1 -> Mux/7
  In8/1 -> Mux/8
  In9/1 -> Mux/9
  In10/1 -> Mux/10
  In11/1 -> Mux/11
  In12/1 -> Mux/12
  In13/1 -> Mux/13
  In14/1 -> Mux/14
  In15/1 -> Mux/15
  In16/1 -> Mux/16
  In17/1 -> Mux/17
  In18/1 -> Mux/18
  In19/1 -> Mux/19
  In20/1 -> Mux/20
  In21/1 -> Mux/21

== system clusterDemo/Cluster1/Cluster2 ==
  In1 : Inport  OutDataType=fixdt(1, 16)  OutScaling=2^0
  In2 : Inport  Port=2
  In3 : Inport  Port=3
  In4 : Inport  Port=4
  In5 : Inport  Port=5
  In6 : Inport  Port=6
  In7 : Inport  Port=7
  In8 : Inport  Port=8
  In9 : Inport  Port=9
  In10 : Inport  Port=10
  In11 : Inport  Port=11
  In12 : Inport  Port=12
  In13 : Inport  Port=13
  In14 : Inport  Port=14
  In15 : Inport  Port=15
  In16 : Inport  Port=16
  In17 : Inport  Port=17
  In18 : Inport  Port=18
  In19 : Inport  Port=19
  In20 : Inport  Port=20
  In21 : Inport  Port=21
  Mux : Mux  Inputs=21
  Scope1 : Scope
      settings: TimeRange=0.5847953216374258  YMin=-0.1657458563535892  YMax=1.21546961325967
  State-Space : StateSpace  A=A  B=B  C=C  D=D  X0=x0+var*rand(1)
  Out1 : Outport  OutDataType=fixdt(1, 16)  OutScaling=2^0
  wires:
  Mux/1 -> State-Space/1
  In1/1 -> Mux/1
  State-Space/1 -> Out1/1, Scope1/1
  In2/1 -> Mux/2
  In3/1 -> Mux/3
  In4/1 -> Mux/4
  In5/1 -> Mux/5
  In6/1 -> Mux/6
  In7/1 -> Mux/7
  In8/1 -> Mux/8
  In9/1 -> Mux/9
  In10/1 -> Mux/10
  In11/1 -> Mux/11
  In12/1 -> Mux/12
  In13/1 -> Mux/13
  In14/1 -> Mux/14
  In15/1 -> Mux/15
  In16/1 -> Mux/16
  In17/1 -> Mux/17
  In18/1 -> Mux/18
  In19/1 -> Mux/19
  In20/1 -> Mux/20
  In21/1 -> Mux/21

== system clusterDemo/Cluster1/Cluster3 ==
  In1 : Inport  OutDataType=fixdt(1, 16)  OutScaling=2^0
  In2 : Inport  Port=2
  In3 : Inport  Port=3
  In4 : Inport  Port=4
  In5 : Inport  Port=5
  In6 : Inport  Port=6
  In7 : Inport  Port=7
  In8 : Inport  Port=8
  In9 : Inport  Port=9
  In10 : Inport  Port=10
  In11 : Inport  Port=11
  In12 : Inport  Port=12
  In13 : Inport  Port=13
  In14 : Inport  Port=14
  In15 : Inport  Port=15
  In16 : Inport  Port=16
  In17 : Inport  Port=17
  In18 : Inport  Port=18
  In19 : Inport  Port=19
  In20 : Inport  Port=20
  In21 : Inport  Port=21
  Mux : Mux  Inputs=21
  Scope1 : Scope
      settings: TimeRange=0.5847953216374258  YMin=-0.1657458563535892  YMax=1.21546961325967
  State-Space : StateSpace  A=A  B=B  C=C  D=D  X0=x0+var*rand(1)
  Out1 : Outport  OutDataType=fixdt(1, 16)  OutScaling=2^0
  wires:
  Mux/1 -> State-Space/1
  In1/1 -> Mux/1
  State-Space/1 -> Out1/1, Scope1/1
  In2/1 -> Mux/2
  In3/1 -> Mux/3
  In4/1 -> Mux/4
  In5/1 -> Mux/5
  In6/1 -> Mux/6
  In7/1 -> Mux/7
  In8/1 -> Mux/8
  In9/1 -> Mux/9
  In10/1 -> Mux/10
  In11/1 -> Mux/11
  In12/1 -> Mux/12
  In13/1 -> Mux/13
  In14/1 -> Mux/14
  In15/1 -> Mux/15
  In16/1 -> Mux/16
  In17/1 -> Mux/17
  In18/1 -> Mux/18
  In19/1 -> Mux/19
  In20/1 -> Mux/20
  In21/1 -> Mux/21

== system clusterDemo/Cluster1/Cluster4 ==
  In1 : Inport  OutDataType=fixdt(1, 16)  OutScaling=2^0
  In2 : Inport  Port=2
  In3 : Inport  Port=3
  In4 : Inport  Port=4
  In5 : Inport  Port=5
  In6 : Inport  Port=6
  In7 : Inport  Port=7
  In8 : Inport  Port=8
  In9 : Inport  Port=9
  In10 : Inport  Port=10
  In11 : Inport  Port=11
  In12 : Inport  Port=12
  In13 : Inport  Port=13
  In14 : Inport  Port=14
  In15 : Inport  Port=15
  In16 : Inport  Port=16
  In17 : Inport  Port=17
  In18 : Inport  Port=18
  In19 : Inport  Port=19
  In20 : Inport  Port=20
  In21 : Inport  Port=21
  Mux : Mux  Inputs=21
  Scope1 : Scope
      settings: TimeRange=0.5847953216374258  YMin=-0.1657458563535892  YMax=1.21546961325967
  State-Space : StateSpace  A=A  B=B  C=C  D=D  X0=x0+var*rand(1)
  Out1 : Outport  OutDataType=fixdt(1, 16)  OutScaling=2^0
  wires:
  Mux/1 -> State-Space/1
  In1/1 -> Mux/1
  State-Space/1 -> Out1/1, Scope1/1
  In2/1 -> Mux/2
  In3/1 -> Mux/3
  In4/1 -> Mux/4
  In5/1 -> Mux/5
  In6/1 -> Mux/6
  In7/1 -> Mux/7
  In8/1 -> Mux/8
  In9/1 -> Mux/9
  In10/1 -> Mux/10
  In11/1 -> Mux/11
  In12/1 -> Mux/12
  In13/1 -> Mux/13
  In14/1 -> Mux/14
  In15/1 -> Mux/15
  In16/1 -> Mux/16
  In17/1 -> Mux/17
  In18/1 -> Mux/18
  In19/1 -> Mux/19
  In20/1 -> Mux/20
  In21/1 -> Mux/21

== system clusterDemo/Cluster1/Cluster5 ==
  In1 : Inport  OutDataType=fixdt(1, 16)  OutScaling=2^0
  In2 : Inport  Port=2
  In3 : Inport  Port=3
  In4 : Inport  Port=4
  In5 : Inport  Port=5
  In6 : Inport  Port=6
  In7 : Inport  Port=7
  In8 : Inport  Port=8
  In9 : Inport  Port=9
  In10 : Inport  Port=10
  In11 : Inport  Port=11
  In12 : Inport  Port=12
  In13 : Inport  Port=13
  In14 : Inport  Port=14
  In15 : Inport  Port=15
  In16 : Inport  Port=16
  In17 : Inport  Port=17
  In18 : Inport  Port=18
  In19 : Inport  Port=19
  In20 : Inport  Port=20
  In21 : Inport  Port=21
  Mux : Mux  Inputs=21
  Scope1 : Scope
      settings: TimeRange=0.5847953216374258  YMin=-0.1657458563535892  YMax=1.21546961325967
  State-Space : StateSpace  A=A  B=B  C=C  D=D  X0=x0+var*rand(1)
  Out1 : Outport  OutDataType=fixdt(1, 16)  OutScaling=2^0
  wires:
  Mux/1 -> State-Space/1
  In1/1 -> Mux/1
  State-Space/1 -> Out1/1, Scope1/1
  In2/1 -> Mux/2
  In3/1 -> Mux/3
  In4/1 -> Mux/4
  In5/1 -> Mux/5
  In6/1 -> Mux/6
  In7/1 -> Mux/7
  In8/1 -> Mux/8
  In9/1 -> Mux/9
  In10/1 -> Mux/10
  In11/1 -> Mux/11
  In12/1 -> Mux/12
  In13/1 -> Mux/13
  In14/1 -> Mux/14
  In15/1 -> Mux/15
  In16/1 -> Mux/16
  In17/1 -> Mux/17
  In18/1 -> Mux/18
  In19/1 -> Mux/19
  In20/1 -> Mux/20
  In21/1 -> Mux/21

== system clusterDemo/Cluster1/Cluster6 ==
  In1 : Inport  OutDataType=fixdt(1, 16)  OutScaling=2^0
  In2 : Inport  Port=2
  In3 : Inport  Port=3
  In4 : Inport  Port=4
  In5 : Inport  Port=5
  In6 : Inport  Port=6
  In7 : Inport  Port=7
  In8 : Inport  Port=8
  In9 : Inport  Port=9
  In10 : Inport  Port=10
  In11 : Inport  Port=11
  In12 : Inport  Port=12
  In13 : Inport  Port=13
  In14 : Inport  Port=14
  In15 : Inport  Port=15
  In16 : Inport  Port=16
  In17 : Inport  Port=17
  In18 : Inport  Port=18
  In19 : Inport  Port=19
  In20 : Inport  Port=20
  In21 : Inport  Port=21
  Mux : Mux  Inputs=21
  Scope1 : Scope
      settings: TimeRange=0.5847953216374258  YMin=-0.1657458563535892  YMax=1.21546961325967
  State-Space : StateSpace  A=A  B=B  C=C  D=D  X0=x0+var*rand(1)
  Out1 : Outport  OutDataType=fixdt(1, 16)  OutScaling=2^0
  wires:
  Mux/1 -> State-Space/1
  In1/1 -> Mux/1
  State-Space/1 -> Out1/1, Scope1/1
  In2/1 -> Mux/2
  In3/1 -> Mux/3
  In4/1 -> Mux/4
  In5/1 -> Mux/5
  In6/1 -> Mux/6
  In7/1 -> Mux/7
  In8/1 -> Mux/8
  In9/1 -> Mux/9
  In10/1 -> Mux/10
  In11/1 -> Mux/11
  In12/1 -> Mux/12
  In13/1 -> Mux/13
  In14/1 -> Mux/14
  In15/1 -> Mux/15
  In16/1 -> Mux/16
  In17/1 -> Mux/17
  In18/1 -> Mux/18
  In19/1 -> Mux/19
  In20/1 -> Mux/20
  In21/1 -> Mux/21

== system clusterDemo/Cluster1/Cluster7 ==
  In1 : Inport  OutDataType=fixdt(1, 16)  OutScaling=2^0
  In2 : Inport  Port=2
  In3 : Inport  Port=3
  In4 : Inport  Port=4
  In5 : Inport  Port=5
  In6 : Inport  Port=6
  In7 : Inport  Port=7
  In8 : Inport  Port=8
  In9 : Inport  Port=9
  In10 : Inport  Port=10
  In11 : Inport  Port=11
  In12 : Inport  Port=12
  In13 : Inport  Port=13
  In14 : Inport  Port=14
  In15 : Inport  Port=15
  In16 : Inport  Port=16
  In17 : Inport  Port=17
  In18 : Inport  Port=18
  In19 : Inport  Port=19
  In20 : Inport  Port=20
  In21 : Inport  Port=21
  Mux : Mux  Inputs=21
  Scope1 : Scope
      settings: TimeRange=0.5847953216374258  YMin=-0.1657458563535892  YMax=1.21546961325967
  State-Space : StateSpace  A=A  B=B  C=C  D=D  X0=x0+var*rand(1)
  Out1 : Outport  OutDataType=fixdt(1, 16)  OutScaling=2^0
  wires:
  Mux/1 -> State-Space/1
  In1/1 -> Mux/1
  State-Space/1 -> Out1/1, Scope1/1
  In2/1 -> Mux/2
  In3/1 -> Mux/3
  In4/1 -> Mux/4
  In5/1 -> Mux/5
  In6/1 -> Mux/6
  In7/1 -> Mux/7
  In8/1 -> Mux/8
  In9/1 -> Mux/9
  In10/1 -> Mux/10
  In11/1 -> Mux/11
  In12/1 -> Mux/12
  In13/1 -> Mux/13
  In14/1 -> Mux/14
  In15/1 -> Mux/15
  In16/1 -> Mux/16
  In17/1 -> Mux/17
  In18/1 -> Mux/18
  In19/1 -> Mux/19
  In20/1 -> Mux/20
  In21/1 -> Mux/21

== system clusterDemo/Cluster1/Cluster8 ==
  In1 : Inport  OutDataType=fixdt(1, 16)  OutScaling=2^0
  In2 : Inport  Port=2
  In3 : Inport  Port=3
  In4 : Inport  Port=4
  In5 : Inport  Port=5
  In6 : Inport  Port=6
  In7 : Inport  Port=7
  In8 : Inport  Port=8
  In9 : Inport  Port=9
  In10 : Inport  Port=10
  In11 : Inport  Port=11
  In12 : Inport  Port=12
  In13 : Inport  Port=13
  In14 : Inport  Port=14
  In15 : Inport  Port=15
  In16 : Inport  Port=16
  In17 : Inport  Port=17
  In18 : Inport  Port=18
  In19 : Inport  Port=19
  In20 : Inport  Port=20
  In21 : Inport  Port=21
  Mux : Mux  Inputs=21
  Scope1 : Scope
      settings: TimeRange=0.5847953216374258  YMin=-0.1657458563535892  YMax=1.21546961325967
  State-Space : StateSpace  A=A  B=B  C=C  D=D  X0=x0+var*rand(1)
  Out1 : Outport  OutDataType=fixdt(1, 16)  OutScaling=2^0
  wires:
  Mux/1 -> State-Space/1
  In1/1 -> Mux/1
  State-Space/1 -> Out1/1, Scope1/1
  In2/1 -> Mux/2
  In3/1 -> Mux/3
  In4/1 -> Mux/4
  In5/1 -> Mux/5
  In6/1 -> Mux/6
  In7/1 -> Mux/7
  In8/1 -> Mux/8
  In9/1 -> Mux/9
  In10/1 -> Mux/10
  In11/1 -> Mux/11
  In12/1 -> Mux/12
  In13/1 -> Mux/13
  In14/1 -> Mux/14
  In15/1 -> Mux/15
  In16/1 -> Mux/16
  In17/1 -> Mux/17
  In18/1 -> Mux/18
  In19/1 -> Mux/19
  In20/1 -> Mux/20
  In21/1 -> Mux/21

== system clusterDemo/Cluster1/Cluster9 ==
  In1 : Inport  OutDataType=fixdt(1, 16)  OutScaling=2^0
  In2 : Inport  Port=2
  In3 : Inport  Port=3
  In4 : Inport  Port=4
  In5 : Inport  Port=5
  In6 : Inport  Port=6
  In7 : Inport  Port=7
  In8 : Inport  Port=8
  In9 : Inport  Port=9
  In10 : Inport  Port=10
  In11 : Inport  Port=11
  In12 : Inport  Port=12
  In13 : Inport  Port=13
  In14 : Inport  Port=14
  In15 : Inport  Port=15
  In16 : Inport  Port=16
  In17 : Inport  Port=17
  In18 : Inport  Port=18
  In19 : Inport  Port=19
  In20 : Inport  Port=20
  In21 : Inport  Port=21
  Mux : Mux  Inputs=21
  Scope1 : Scope
      settings: TimeRange=0.5847953216374258  YMin=-0.1657458563535892  YMax=1.21546961325967
  State-Space : StateSpace  A=A  B=B  C=C  D=D  X0=x0+var*rand(1)
  Out1 : Outport  OutDataType=fixdt(1, 16)  OutScaling=2^0
  wires:
  Mux/1 -> State-Space/1
  In1/1 -> Mux/1
  State-Space/1 -> Out1/1, Scope1/1
  In2/1 -> Mux/2
  In3/1 -> Mux/3
  In4/1 -> Mux/4
  In5/1 -> Mux/5
  In6/1 -> Mux/6
  In7/1 -> Mux/7
  In8/1 -> Mux/8
  In9/1 -> Mux/9
  In10/1 -> Mux/10
  In11/1 -> Mux/11
  In12/1 -> Mux/12
  In13/1 -> Mux/13
  In14/1 -> Mux/14
  In15/1 -> Mux/15
  In16/1 -> Mux/16
  In17/1 -> Mux/17
  In18/1 -> Mux/18
  In19/1 -> Mux/19
  In20/1 -> Mux/20
  In21/1 -> Mux/21

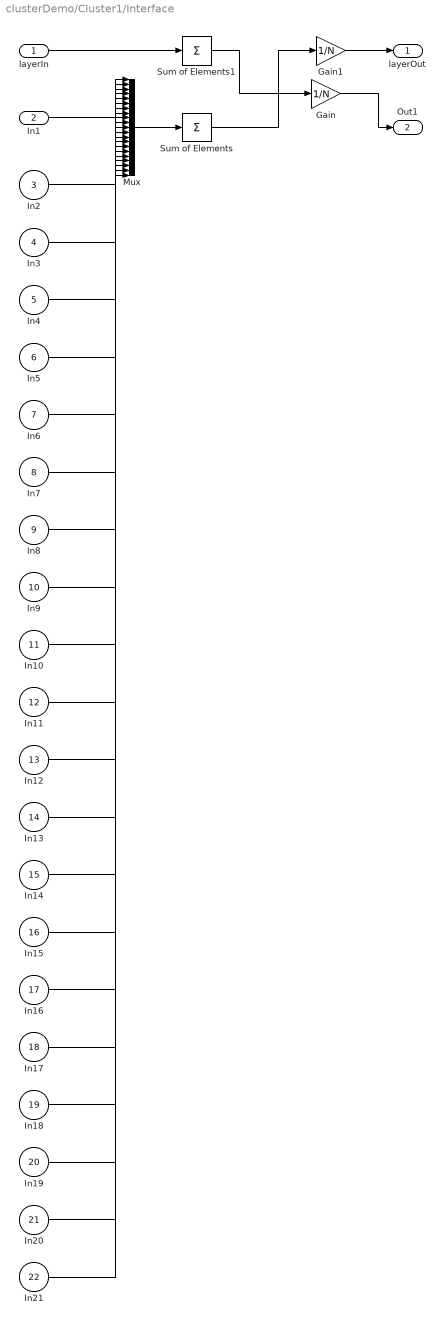
== system clusterDemo/Cluster1/Interface ==
  layerIn : Inport  OutDataType=fixdt(1, 16)  OutScaling=2^0
  In1 : Inport  Port=2  OutDataType=fixdt(1, 16)  OutScaling=2^0
  In2 : Inport  Port=3
  In3 : Inport  Port=4
  In4 : Inport  Port=5
  In5 : Inport  Port=6
  In6 : Inport  Port=7
  In7 : Inport  Port=8
  In8 : Inport  Port=9
  In9 : Inport  Port=10
  In10 : Inport  Port=11
  In11 : Inport  Port=12
  In12 : Inport  Port=13
  In13 : Inport  Port=14
  In14 : Inport  Port=15
  In15 : Inport  Port=16
  In16 : Inport  Port=17
  In17 : Inport  Port=18
  In18 : Inport  Port=19
  In19 : Inport  Port=20
  In20 : Inport  Port=21
  In21 : Inport  Port=22
  Gain : Gain  Gain=1/N  ParameterDataType=fixdt(1, 16)  ParameterScaling=2^0  OutDataType=fixdt(1, 16)  OutScaling=2^0
  Gain1 : Gain  Gain=1/N  ParameterDataType=fixdt(1, 16)  ParameterScaling=2^0  OutDataType=fixdt(1, 16)  OutScaling=2^0
  Mux : Mux  Inputs=21
  Sum of Elements : Sum  Inputs=+  OutDataType=fixdt(1, 16)  OutScaling=2^-10
  Sum of Elements1 : Sum  Inputs=+  OutDataType=fixdt(1, 16)  OutScaling=2^-10
  layerOut : Outport  OutDataType=fixdt(1, 16)  OutScaling=2^0
  Out1 : Outport  Port=2  OutDataType=fixdt(1, 16)  OutScaling=2^0
  wires:
  Mux/1 -> Sum of Elements/1
  In1/1 -> Mux/1
  Sum of Elements/1 -> Gain1/1
  layerIn/1 -> Sum of Elements1/1
  Sum of Elements1/1 -> Gain/1
  Gain/1 -> Out1/1
  Gain1/1 -> layerOut/1
  In2/1 -> Mux/2
  In3/1 -> Mux/3
  In4/1 -> Mux/4
  In5/1 -> Mux/5
  In6/1 -> Mux/6
  In7/1 -> Mux/7
  In8/1 -> Mux/8
  In9/1 -> Mux/9
  In10/1 -> Mux/10
  In11/1 -> Mux/11
  In12/1 -> Mux/12
  In13/1 -> Mux/13
  In14/1 -> Mux/14
  In15/1 -> Mux/15
  In16/1 -> Mux/16
  In17/1 -> Mux/17
  In18/1 -> Mux/18
  In19/1 -> Mux/19
  In20/1 -> Mux/20
  In21/1 -> Mux/21

== system clusterDemo/Cluster2/Cluster ==
  In1 : Inport  OutDataType=fixdt(1, 16)  OutScaling=2^0
  In2 : Inport  Port=2
  In3 : Inport  Port=3
  In4 : Inport  Port=4
  In5 : Inport  Port=5
  In6 : Inport  Port=6
  In7 : Inport  Port=7
  In8 : Inport  Port=8
  In9 : Inport  Port=9
  In10 : Inport  Port=10
  In11 : Inport  Port=11
  In12 : Inport  Port=12
  In13 : Inport  Port=13
  In14 : Inport  Port=14
  In15 : Inport  Port=15
  In16 : Inport  Port=16
  In17 : Inport  Port=17
  In18 : Inport  Port=18
  In19 : Inport  Port=19
  In20 : Inport  Port=20
  In21 : Inport  Port=21
  Mux : Mux  Inputs=21
  Scope1 : Scope
      settings: TimeRange=0.5847953216374258  YMin=-0.1657458563535892  YMax=1.21546961325967
  State-Space : StateSpace  A=A  B=B  C=C  D=D  X0=x0+var*rand(1)
  Out1 : Outport  OutDataType=fixdt(1, 16)  OutScaling=2^0
  wires:
  Mux/1 -> State-Space/1
  In1/1 -> Mux/1
  State-Space/1 -> Out1/1, Scope1/1
  In2/1 -> Mux/2
  In3/1 -> Mux/3
  In4/1 -> Mux/4
  In5/1 -> Mux/5
  In6/1 -> Mux/6
  In7/1 -> Mux/7
  In8/1 -> Mux/8
  In9/1 -> Mux/9
  In10/1 -> Mux/10
  In11/1 -> Mux/11
  In12/1 -> Mux/12
  In13/1 -> Mux/13
  In14/1 -> Mux/14
  In15/1 -> Mux/15
  In16/1 -> Mux/16
  In17/1 -> Mux/17
  In18/1 -> Mux/18
  In19/1 -> Mux/19
  In20/1 -> Mux/20
  In21/1 -> Mux/21

== system clusterDemo/Cluster2/Cluster1 ==
  In1 : Inport  OutDataType=fixdt(1, 16)  OutScaling=2^0
  In2 : Inport  Port=2
  In3 : Inport  Port=3
  In4 : Inport  Port=4
  In5 : Inport  Port=5
  In6 : Inport  Port=6
  In7 : Inport  Port=7
  In8 : Inport  Port=8
  In9 : Inport  Port=9
  In10 : Inport  Port=10
  In11 : Inport  Port=11
  In12 : Inport  Port=12
  In13 : Inport  Port=13
  In14 : Inport  Port=14
  In15 : Inport  Port=15
  In16 : Inport  Port=16
  In17 : Inport  Port=17
  In18 : Inport  Port=18
  In19 : Inport  Port=19
  In20 : Inport  Port=20
  In21 : Inport  Port=21
  Mux : Mux  Inputs=21
  Scope1 : Scope
      settings: TimeRange=0.5847953216374258  YMin=-0.1657458563535892  YMax=1.21546961325967
  State-Space : StateSpace  A=A  B=B  C=C  D=D  X0=x0+var*rand(1)
  Out1 : Outport  OutDataType=fixdt(1, 16)  OutScaling=2^0
  wires:
  Mux/1 -> State-Space/1
  In1/1 -> Mux/1
  State-Space/1 -> Out1/1, Scope1/1
  In2/1 -> Mux/2
  In3/1 -> Mux/3
  In4/1 -> Mux/4
  In5/1 -> Mux/5
  In6/1 -> Mux/6
  In7/1 -> Mux/7
  In8/1 -> Mux/8
  In9/1 -> Mux/9
  In10/1 -> Mux/10
  In11/1 -> Mux/11
  In12/1 -> Mux/12
  In13/1 -> Mux/13
  In14/1 -> Mux/14
  In15/1 -> Mux/15
  In16/1 -> Mux/16
  In17/1 -> Mux/17
  In18/1 -> Mux/18
  In19/1 -> Mux/19
  In20/1 -> Mux/20
  In21/1 -> Mux/21

== system clusterDemo/Cluster2/Cluster10 ==
  In1 : Inport  OutDataType=fixdt(1, 16)  OutScaling=2^0
  In2 : Inport  Port=2
  In3 : Inport  Port=3
  In4 : Inport  Port=4
  In5 : Inport  Port=5
  In6 : Inport  Port=6
  In7 : Inport  Port=7
  In8 : Inport  Port=8
  In9 : Inport  Port=9
  In10 : Inport  Port=10
  In11 : Inport  Port=11
  In12 : Inport  Port=12
  In13 : Inport  Port=13
  In14 : Inport  Port=14
  In15 : Inport  Port=15
  In16 : Inport  Port=16
  In17 : Inport  Port=17
  In18 : Inport  Port=18
  In19 : Inport  Port=19
  In20 : Inport  Port=20
  In21 : Inport  Port=21
  Mux : Mux  Inputs=21
  Scope1 : Scope
      settings: TimeRange=0.5847953216374258  YMin=-0.1657458563535892  YMax=1.21546961325967
  State-Space : StateSpace  A=A  B=B  C=C  D=D  X0=x0+var*rand(1)
  Out1 : Outport  OutDataType=fixdt(1, 16)  OutScaling=2^0
  wires:
  Mux/1 -> State-Space/1
  In1/1 -> Mux/1
  State-Space/1 -> Out1/1, Scope1/1
  In2/1 -> Mux/2
  In3/1 -> Mux/3
  In4/1 -> Mux/4
  In5/1 -> Mux/5
  In6/1 -> Mux/6
  In7/1 -> Mux/7
  In8/1 -> Mux/8
  In9/1 -> Mux/9
  In10/1 -> Mux/10
  In11/1 -> Mux/11
  In12/1 -> Mux/12
  In13/1 -> Mux/13
  In14/1 -> Mux/14
  In15/1 -> Mux/15
  In16/1 -> Mux/16
  In17/1 -> Mux/17
  In18/1 -> Mux/18
  In19/1 -> Mux/19
  In20/1 -> Mux/20
  In21/1 -> Mux/21

== system clusterDemo/Cluster2/Cluster11 ==
  In1 : Inport  OutDataType=fixdt(1, 16)  OutScaling=2^0
  In2 : Inport  Port=2
  In3 : Inport  Port=3
  In4 : Inport  Port=4
  In5 : Inport  Port=5
  In6 : Inport  Port=6
  In7 : Inport  Port=7
  In8 : Inport  Port=8
  In9 : Inport  Port=9
  In10 : Inport  Port=10
  In11 : Inport  Port=11
  In12 : Inport  Port=12
  In13 : Inport  Port=13
  In14 : Inport  Port=14
  In15 : Inport  Port=15
  In16 : Inport  Port=16
  In17 : Inport  Port=17
  In18 : Inport  Port=18
  In19 : Inport  Port=19
  In20 : Inport  Port=20
  In21 : Inport  Port=21
  Mux : Mux  Inputs=21
  Scope1 : Scope
      settings: TimeRange=0.5847953216374258  YMin=-0.1657458563535892  YMax=1.21546961325967
  State-Space : StateSpace  A=A  B=B  C=C  D=D  X0=x0+var*rand(1)
  Out1 : Outport  OutDataType=fixdt(1, 16)  OutScaling=2^0
  wires:
  Mux/1 -> State-Space/1
  In1/1 -> Mux/1
  State-Space/1 -> Out1/1, Scope1/1
  In2/1 -> Mux/2
  In3/1 -> Mux/3
  In4/1 -> Mux/4
  In5/1 -> Mux/5
  In6/1 -> Mux/6
  In7/1 -> Mux/7
  In8/1 -> Mux/8
  In9/1 -> Mux/9
  In10/1 -> Mux/10
  In11/1 -> Mux/11
  In12/1 -> Mux/12
  In13/1 -> Mux/13
  In14/1 -> Mux/14
  In15/1 -> Mux/15
  In16/1 -> Mux/16
  In17/1 -> Mux/17
  In18/1 -> Mux/18
  In19/1 -> Mux/19
  In20/1 -> Mux/20
  In21/1 -> Mux/21
